simulink library "etherlab_lib_exp"  (Simulink 7.0)
undefined symbols (not defined in the file or in its folder): Address, catch_check
settings Model: Creator=rich  LastModifiedBy=ab  ExtModeAutoUpdateStatusClock=off

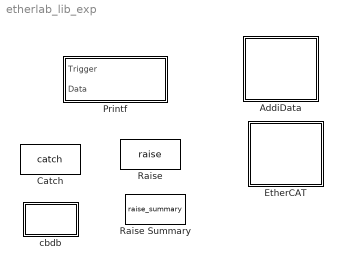
== system etherlab_lib_exp ==
  AddiData : Subsystem
  Catch : S-Function  InitFcn=catch_check(gcb,'CheckIds');  FunctionName=catch  Parameters=ErrId,dtype,Width,TSample  mask{ErrId=E10, dtype=boolean, TSample=0, Width=0, SrcPath=0, SrcCount=0}
      mask prompts: ErrId "Error Identifier"; dtype "Output Data Type Mode"; TSample "Sample Time (-1 inherited)"; SrcPath "Source Paths (Info only)"; SrcCount "Source Count"
      mask StyleString: edit,popup(double|single|int8|uint8|int16|uint16|int32|uint32|boolean|Inherit via back propagation),edit,edit,edit,edit
      mask CallbackString: catch_check(gcb,'CheckIds');|||||
      mask Display: fprintf('%s',ErrId);
  EtherCAT : Subsystem
  Printf : Subsystem  mask{format=0}
      mask prompts: format "Format String"
  Raise : S-Function  FunctionName=raise  Parameters=ErrId,ErrStr,TSample  mask{ErrId=E10, ErrStr=Voltage Too High, TSample=-1, DstPath=0, DstCount=0}
      mask prompts: ErrId "Error Identifier"; ErrStr "Error String"; TSample "Sample Time (-1 inherited)"; DstPath "Destination Paths"; DstCount "Destination Count"
      settings: CopyFcn=raise_check(gcb,'CheckCopy');
      mask CallbackString: raise_check(gcb,'CheckId');||||
      mask Display: fprintf('%s',ErrId);
  Raise Summary : S-Function  FunctionName=raise_summary  Parameters=ErrId,ErrStr,ErrSrc,DstPath  mask{ErrId=E1x, ErrStr=Voltage Too High, ErrSrc=E10, DstPath=0}
      mask prompts: ErrId "Error Identifier"; ErrStr "Error String"; ErrSrc "Error Sources"; DstPath "Destination Paths"
      settings: CopyFcn=raise_summary_check(gcb,'CheckCopy');
      mask Display: fprintf('%s\n%s',ErrId,ErrSrc);
  cbdb : Subsystem  LoadFcn=|  InitFcn=|  StartFcn=|  StopFcn=|  ClipboardFcn=|
      | if ~strcmp(gcs,'rtai_lib')
      | display('LoadFcn');       
      | end
      | if ~strcmp(gcs,'rtai_lib')
      | display('InitFcn');       
      | end
      | if ~strcmp(gcs,'rtai_lib')
      | display('StartFcn');      
      | end
      | if ~strcmp(gcs,'rtai_lib')
      | display('StopFcn');       
      | end
      | if ~strcmp(gcs,'rtai_lib')
      | display('ClipboardFcn');  
      | end
      settings: CopyFcn=|
      | if ~strcmp(gcs,'rtai_lib')
      | display('CopyFcn');
      | end
      settings: DeleteFcn=|
      | if ~strcmp(gcs,'rtai_lib')
      | display('DeleteFcn');
      | end
      settings: UndoDeleteFcn=|
      | if ~strcmp(gcs,'rtai_lib')
      | display('UndoDeleteFcn');
      | end
      settings: ModelCloseFcn=|
      | if ~strcmp(gcs,'rtai_lib')
      | display('ModelCloseFcn');
      | end
      settings: PreSaveFcn=|
      | if ~strcmp(gcs,'rtai_lib')
      | display('PreSaveFcn');
      | end
      settings: PostSaveFcn=|
      | if ~strcmp(gcs,'rtai_lib')
      | display('PostSaveFcn');
      | end
      settings: NameChangeFcn=|
      | if ~strcmp(gcs,'rtai_lib')
      | display('NameChangeFcn');
      | end
      settings: DestroyFcn=|
      | if ~strcmp(gcs,'rtai_lib')
      | display('DestroyFcn');
      | end
      settings: OpenFcn=|
      | if ~strcmp(gcs,'rtai_lib')
      | display('OpenFcn');
      | end
      settings: CloseFcn=|
      | if ~strcmp(gcs,'rtai_lib')
      | display('CloseFcn');
      | end
      settings: ParentCloseFcn=|
      | if ~strcmp(gcs,'rtai_lib')
      | display('ParentCloseFcn');
      | end
      settings: MoveFcn=|
      | if ~strcmp(gcs,'rtai_lib')
      | display('MoveFcn');
      | end
      mask Display: disp('Callback\nDebugger');

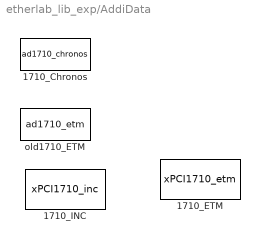
== system etherlab_lib_exp/AddiData ==
  1710_Chronos : S-Function  FunctionName=ad1710_chronos  Parameters=b_BoardHandle,b_ModuleNumber,b_ChronoMode,b_PCIInputClock,b_TimeUnit,ul_TimeOut,b_TimeoutUnit  mask{b_BoardHandle=0, b_ModuleNumber=0, b_ChronoMode=0, b_PCIInputClock=30MHz, b_TimeUnit=Microseconds, ul_TimeOut=0, b_TimeoutUnit=Micoseconds}
      mask prompts: b_BoardHandle "Board Handle"; b_ModuleNumber "Module Number"; b_ChronoMode "Chrono Mode"; b_PCIInputClock "PCI Input Clock"; b_TimeUnit "Time Unit"; ul_TimeOut "Timeout"; b_TimeoutUnit "Timeout Unit"
      mask StyleString: edit,popup(0|1|2|3),popup(0|1|2|3|4|5|6|7),popup(30MHz|33MHz|40MHz),popup(Nanoseconds|Microseconds|Milliseconds|Seconds|Minutes),edit,popup(Nanoseconds|Micoseconds|Milliseconds|Seconds|Minutes)
      mask Display:
      | fprintf('1710 Chrono\nB:%i M/d:%i',
      | b_BoardHandle,b_ModuleNumber);
  1710_ETM : S-Function  FunctionName=xPCI1710_etm  Parameters=device,module,clock_src,divisor,op_type,tsample  mask(Addi Data 1710 ETM){device=01:0A, module=0, clock_src=Internal 40MHz, divisor=1, op_type=double, scale=0, offset=0, tsample=0}
      mask prompts: device "PCI Device"; module "Module Number"; clock_src "Clock Source"; divisor "Clock Divisor"; op_type "Output Data Type"; scale "Output Full Scale"; offset "Output Offset"; tsample "Sampling Time (-1 inherited)"
      mask help: This block implements the Edge Triggered Timer Mode for the 1710 Addi Data timer card.
      mask init:
      | device = test_var(device);
      mask StyleString: edit,popup(0|1|2|3),popup(Internal 40MHz|PCI Bus 33/30Mhz),edit,popup(double|single|int8|uint8|int16|uint16|int32|uint32|boolean|Inherited via back propagation),edit,edit,edit
      mask Display:
      | fprintf('xPCI1710 ETM\nPCI: %s\nModule: %i',
      | device,module-1);
  1710_INC : S-Function  FunctionName=xPCI1710_inc  Parameters=device,module,mode,width,op_type,preset,tsample  mask(Addi Data 1710 INC){device=03:0E, module=0, mode=Quadruple, width=32-Bit, op_type=double, preset=off, tsample=0}
      mask prompts: device "PCI Device"; module "Module Number"; width "Counter Width"; op_type "Output Data Type"; preset "Preset Input"; tsample "Sampling Time (-1 inherited)"
      mask help: This block implements the Incremental Counter Mode for the 1710 Addi Data timer card.
      mask init:
      | device = test_var(device);
      mask StyleString: edit,popup(0|1|2|3),popup(Quadruple|Double|Simple|Direct),popup(32-Bit|16-Bit),popup(double|single|int8|uint8|int16|uint16|int32|uint32|boolean|Inherited via back propagation),checkbox,edit
      mask Display:
      | fprintf('xPCI1710 INC\nPCI: %s\nModule: %i',
      | device,module-1);
  old1710_ETM : S-Function  FunctionName=ad1710_etm  Parameters=b_BoardHandle,b_ModuleNumber,b_ClockSelection,b_TimingUnit,ul_Timing  mask(Addi Data 1710 ETM){b_BoardHandle=0, b_ModuleNumber=0, b_ClockSelection=PCI 30MHz, b_TimingUnit=Microseconds, ul_Timing=0}
      mask prompts: b_BoardHandle "Board Handle"; b_ModuleNumber "Module Number"; b_ClockSelection "Clock Selection"; b_TimingUnit "Timing Unit"; ul_Timing "Time Base"
      mask help:
      | This block implements the Edge Triggered Mode for the 1710 Addi Data timer card.
      |
      | Both counters are exported as a vector.
      mask StyleString: edit,popup(0|1|2|3),popup(PCI 30MHz|PCI 33MHz|Internal 40MHz),popup(Nanoseconds|Microseconds|Milliseconds),edit
      mask Display:
      | fprintf('1710 ETM\nB:%i M/d:%i',
      | b_BoardHandle,b_ModuleNumber);

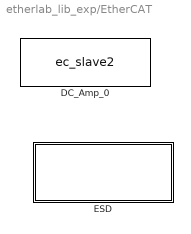
== system etherlab_lib_exp/EtherCAT ==
  DC_Amp_0 : S-Function  FunctionName=ec_slave2  Parameters=Address,config.SlaveConfig,config.SdoConfig,config.SoeConfig,config.IO,debug,tsample  mask(EL73x2){master=0, index=1, model=EL7332r00100000, dcmode=FreeRun/SM-Synchron, dccustom=[1 hex2dec('700') 0 0 0 0 0 0 0], max_current=[0 0], nom_current=[0 0], nom_volt=[0 0], resistance=[0 0], red_current_neg=[0 0], red_current_pos=[0 0], kp=[200 200], ki=[2 2], voltage_adjust_ch1=off, voltage_adjust_ch2=off, current_adjust_ch1=off, current_adjust_ch2=off, op_mode_ch1=Velocity direct, op_mode_ch2=Velocity direct, inv_dir_ch1=off, inv_dir_ch2=off, show_info_channels=off, datafield1_ch1=Coil Voltage, datafield2_ch1=Coil Current, datafield1_ch2=Coil Voltage, datafield2_ch2=Coil Current, show_digital_inputs=off, inv_input1_ch1=off, inv_input2_ch1=off, inv_input1_ch2=off, inv_input2_ch2=off, mode_input1_ch1=Normal Input, mode_input2_ch1=Normal Input, mode_input1_ch2=Normal Input, mode_input2_ch2=Normal Input, tsample=-1, debug=0, updatefcn=beckhoff_el73x2}
      mask prompts: index "Slave Index"; model "Device Model"; dcmode "DC Mode"; dccustom "DC Customized"; max_current "Max Motor Current in mA"; nom_current "Nominal Motor Currnet in mA"; nom_volt "Nominal Motor Voltage in mV"; resistance "Motor Resistance in 1/100 Ohm"; red_current_neg "Reduced Current (negative) in mA"; red_current_pos "Reduced Current (positive) in mA"; kp "Controller kp"; ki "Controller ki"; voltage_adjust_ch1 "Enable Voltage Adjustment Channel1"; voltage_adjust_ch2 "Enable Voltage Adjustment Channel2"; current_adjust_ch1 "Enable Current Adjustment Channel1"; current_adjust_ch2 "Enable Current Adjustment Channel2"; op_mode_ch1 "Operating Mode Channel1"; op_mode_ch2 "Operating Mode Channel2"; inv_dir_ch1 "Invert Motor direction Channel1"; inv_dir_ch2 "Invert Motor direction Channel2"; show_info_channels "Show Info Fields"; datafield1_ch1 "Info Field1 Channel 1"; datafield2_ch1 "Info Field2 Channel 2"; datafield1_ch2 "Info Field1 Channel 2"; datafield2_ch2 "Info Field2 Channel 2"; show_digital_inputs "Show Digital Inputs"; inv_input1_ch1 "Invert DI1 Channel1"; inv_input2_ch1 "Invert DI2 Channel1"; inv_input1_ch2 "Invert DI1 Channel2"; inv_input2_ch2 "Invert DI2 Channel2"; mode_input1_ch1 "Mode DI1 Channel1"; mode_input2_ch1 "Mode DI2 Channel1"; mode_input1_ch2 "Mode DI1 Channel2"; mode_input2_ch2 "Mode DI2 Channel2"; tsample "Sample Time (-1 for inherited)"
      mask help: Beckhoff 2 Channel DC Amplifier EL73x2
      mask init:
      | masterStr = '';
      | positionStr = '';
      | 
      | [Address masterStr positionStr] = getEtherCATAddress(gcb,master,index);
      | 
      | selection = beckhoff_el73x2('getmodel',model);
      | if isempty(selection)
      |     return;
      | end
      | 
      | func = selection{3};
      | 
      | device = beckhoff_el73x2('loaddescription',selection);
      | if isempty(device)
      |    return; 
      | end
      | 
      | 
      | %Prepare S-Funtion structure
      | 
      | config = beckhoff_el73x2('process',selection,device, ...
      |         max_current,nom_current,nom_volt,resistance, ...
      |         red_current_neg,red_current_pos, kp,ki,...
      |         voltage_adjust_ch1,current_adjust_ch1,...
      |         op_mode_ch1, inv_dir_ch1, ...
      |         datafield1_ch1,datafield2_ch1, ...
      |         inv_input1_ch1, inv_input2_ch1,...
      |         mode_input1_ch1, mode_input2_ch1,...
      |         voltage_adjust_ch2,current_adjust_ch2,...
      |         op_mode_ch2, inv_dir_ch2, ...
      |         datafield1_ch2,datafield2_ch2, ...
      |         inv_input1_ch2, inv_input2_ch2,...
      |         mode_input1_ch2, mode_input2_ch2,...
      |        show_digital_inputs, show_info_channels,...
      |        dcmode,dccustom ...
      |     );
      mask Help:
      | This block implements the EtherCAT 2 Channel DC Amplifier Terminal EL73x2.
      | <p/>
      | The block input and output depends generally on the configured functionality. Please read the Terminal documentation.
      | <p/>
      | The following Terminals are supported:
      | <center>
      | <table width="80%">
      | <tr><td>EL7332</td><td></td></tr>
      | </table>
      | </center>
      | <p/>
      | 
      | 
      | 
      | <h4>Inputs:</h4>
      | Every Block Input is a 2-element Vector ([Channel1 Channel2])
      | <p>
      | Following Inputs exists:
      | <ul>
      | <li> Enable</li>
      | <li> Reset</li>
      | <li> Reduce Torque</li>
      | <li> Setpoint Current</li>
      | <ul/>
      | <h4>Outputs:</h4>
      | Every Block Output is a 2-element Vector ([Channel1 Channel2])
      | <p>
      | Following Outputs exists:
      | <ul>
      | <li> Ready to Enable </li>
      | <li> Ready </li>
      | <li> Warning</li>
      | <li> Error</li>
      | <li> Digital Input 1 (optional)</li>
      | <li> Digital Input 2 (optional)</li>
      | <li> Info Channel 1 (optional)</li>
      | <li> Info Channel 2 (optional)</li>
      | </ul>
      | Choose and set the following options:
      | <h4>Master:</h4>
      | Set the EtherCAT Master of this terminal.
      | 
      | <h4>Slave Index:</h4>
      | Set the EtherCAT slave index. Following address formats are allowed:
      | <ol>
      | <li> Absolute addressing: a scalar number <<b><tt>n</tt></b>> representing the (zero based) absolute position in the bus.
      | <li> SSId addressing: the Secondary Slave (or 'Alias') Addressing has the form <<b><tt>[alias position]</tt></b>> where <b><tt>alias</tt></b> is the Secondary Slave Id of the EtherCAT slave and <b><tt>position</tt></b> is the offset after the slave with the given <b><tt>alias</tt></b>. The SSId has to be preprogrammed into the slave with other service tools (see 'ethercat alias --help').
      | </ol>
      | 
      | <h4>Device Model:</h4>
      | Choose the device at the Indexed position of the master.
      | 
      | <h4>DC Mode:</h4>
      | Choose the DC Mode for the module.
      | 
      | <h4>DC Customer:</h4>
      | Do customized DC Settings in a vector
      | <<b><tt>[Index AssignActivate cycletimesync0 factor0 cycletimeshift0 input0 cycletimesync1 factor1 cylcetimeshift1]</tt></b>>
      | 
      | <ul>
      | <li><<b><tt>Index:</tt></b>> preload index from XML desctiption, to get the oversampling configuration from an existing DC-mode.
      | <li><<b><tt>AssignActivate:</tt></b>> Value for DC-mode setting
      | <li><<b><tt>cycletimesync0:</tt></b>> CycletimeSync0 Value
      | <li><<b><tt>factor0:</tt></b>> 1 or 0. If factor0 equals one the cycletimesync0 value is internally set to the process cycletime.
      | <li><<b><tt>cycletimeshift0:</tt></b>> Cycletimeshift0 Value
      | <li><<b><tt>input0:</tt></b>> 1 or 0. If inpot0 equals one the Slave is synced on the input event
      | <li><<b><tt>cycletimesync1:</tt></b>> CycletimeSync1 Value
      | <li><<b><tt>factor1:</tt></b>> 1 or 0. If factor1 equals one the cycletimesync1 value is internally set to the process cycletime.
      | <li><<b><tt>cylcetimeshift1:</tt></b>> Cycletimeshift1 Value
      | </ul>
      | 
      | <h4>Max Motor Current in mA:</h4>
      | Maximal Motor Current in mA. Value has to be a 2 element vector: [0 0] ([Channel1 Channe2])
      | 
      | <h4>Nominal Motor Current in mA:</h4>
      | Nominal Motor Current in mA. Value has to be a 2 element vector: [0 0] ([Channel1 Channe2])
      | 
      | <h4>Nominal Motor Voltage in mV:</h4>
      | Nominal Motor Voltage in mV. Value has to be a 2 element vector: [0 0] ([Channel1 Channe2])
      | 
      | <h4>Motor Resistance in 1/100 Ohm:</h4>
      | Motor Resistance in 1/100 Ohm. Value has to be a 2 element vector: [0 0] ([Channel1 Channe2])
      | 
      | <h4>Reduced Current (negative) in mA:</h4>
      | Reduced Current Value in negative Direction. Value has to be a 2 element vector: [0 0] ([Channel1 Channe2])
      | 
      | <h4>Reduced Current (positive) in mA:</h4>
      | Reduced Current Value in positive Direction. Value has to be a 2 element vector: [0 0] ([Channel1 Channe2])
      | 
      | <h4>Controller kp:</h4>
      | Motor Controller Setting for kp. Value has to be a 2 element vector: [0 0] ([Channel1 Channe2])
      | 
      | <h4>Controller ki:</h4>
      | Motor Controller Setting for ki. Value has to be a 2 element vector: [0 0] ([Channel1 Channe2])
      | 
      | <h4>Enable Voltage Adjustment Channel[1,2]:</h4>
      | Activates Voltage swing compensation for Channel [1,2].
      | 
      | <h4>Enable Current Adjustment Channel[1,2]:</h4>
      | Activates RxI compensation for Channel [1,2].
      | 
      | <h4>Operating Mode Channel[1,2]:</h4>
      | Select Operating Mode for Channel [1,2]. Actually only Velocity direct is implemeneted.
      | 
      | <h4>Invert Motor direction Channel[1,2]:</h4>
      | Invert Rotyting direction for Channel [1,2].
      | 
      | <h4>Show Info Fields:</h4>
      | Enable or Disable the Output of the configurable PDO Outputs.
      | 
      | <h4>Info Field[X=1,2] Channel[Y=1,2]</h4>
      | Configure the output info fields. 2 Info outputs per channel exists.
      | Actually only the selection of State, Current and Voltage are supported.
      | 
      | <h4>Show Digital Inputs:</h4>
      | Enable or Disable the Output of the digital inputs.
      | 
      | <h4>Invert DI[X=1,2] Channel[Y=1,2]</h4>
      | Invert the digital input. 2  digital inputs per channel exists.
      | 
      | <h4>Mode DI[X=1,2] Channel[Y=1,2]</h4>
      | Working mode of the digital input. 2  digital inputs per channel exists.
      | Normal input or Hardware enable are available.
      | 
      | <p>
      | To get further information for parameter configuration, please read the terminal documentation.
      | <p>
      | Set the <b>Sample Time</b> for the block. <tt>0</tt> is continuous sample time (runs at the model's base rate). Setting <tt>-1</tt> will try to set the time using back propagation.
      mask StyleString: edit,edit,popup(EL7332r00100000|EL7332r00110000),popup(FreeRun/SM-Synchron|DC-Synchron|DC-Customized),edit,edit,edit,edit,edit,edit,edit,edit,edit,checkbox,checkbox,checkbox,checkbox,popup(Automatic|Velocity direct|Velocity controller|Position controller),popup(Automatic|Velocity direct|Velocity controller|Position controller),checkbox,checkbox,checkbox,popup(Status word|Coil Voltage|Coil Current),popup(Status word|Coil Voltage|Coil Current),popup(Status word|Coil Voltage|Coil Current),popup(Status word|Coil Voltage|Coil Current),checkbox,checkbox,checkbox,checkbox,checkbox,popup(Normal Input|Hardware Enable),popup(Normal Input|Hardware Enable),popup(Normal Input|Hardware Enable),popup(Normal Input|Hardware Enable),edit,edit,edit
      mask CallbackString: ||beckhoff_el73x2('model');|beckhoff_el73x2('dc');||||||||||||||||||||||||||||||||||
      mask Display:
      | fprintf('%s\n%s \nM:%s Idx:%s',...
      |     model,func,masterStr,positionStr)
  ESD : Subsystem
      mask Display: image(imread('ESD.png'))

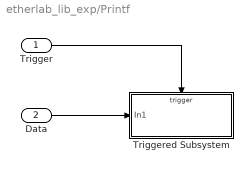
== system etherlab_lib_exp/Printf ==
  Trigger : Inport  OutDataType=sfix(16)  OutScaling=2^0
  Data : Inport  Port=2  OutDataType=sfix(16)  OutScaling=2^0
  Triggered Subsystem : Subsystem  TreatAsAtomicUnit=on
  wires:
  Trigger/1 -> Triggered Subsystem/Trigger
  Data/1 -> Triggered Subsystem/1(In1)

== system etherlab_lib_exp/cbdb ==

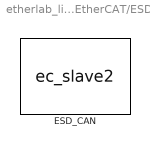
== system etherlab_lib_exp/EtherCAT/ESD ==
  ESD_CAN : S-Function  FunctionName=ec_slave2  Parameters=Address,conf.SlaveConfig,conf.SdoConfig,conf.SoeConfig,conf.IO,debug,tsample  mask(ESD EtherCAT CAN Gateway){master=0, index=1, model=CANr00000000, numberrx=1, numbertx=1, isext=off, baudrate=500, rxfilter=[], nodeadr=1, tsample=-1, debug=0, updatefcn=esd_cangateway}
      mask prompts: index "Slave Index"; model "Device Model"; numberrx "MailboxSize RX"; numbertx "MailboxSize TX"; isext "Extended ID"; baudrate "Baudrate in kBit/s"; rxfilter "RX Filter IDs"; nodeadr "Node ID"; tsample "Sample Time (-1 for inherited)"
      mask help:
      | ESD EtherCAT
      | CAN Gateway
      mask init:
      | masterStr = '';
      | positionStr = '';
      | [Address masterStr positionStr] = getEtherCATAddress(gcb,master,index);
      | 
      | selection = esd_cangateway('getmodel',model);
      | if isempty(selection)
      |     return;
      | end
      | 
      | func = selection{3};
      | 
      | device = esd_cangateway('loaddescription',selection);
      | if isempty(device)
      |    return; 
      | end
      | 
      | 
      | %Prepare S-Funtion structure
      | 
      | conf = esd_cangateway('process',selection,device,numberrx,numbertx,isext,baudrate,rxfilter,nodeadr);
      mask Help:
      | This block generically implements the ESD EtherCAT CAN Gateway.
      | 
      | <p/>
      | The following Terminals are supported:
      | <center>
      | <table width="80%">
      | <tr><td>CAN</td><td> EtherCAT CAN Gateway</td></tr>
      | </table>
      | </center>
      | <h3> Inputs / Outputs</h3>
      | <h4>Inputs</h4>
      | There are two block inputs.
      | <p>
      | First port the static informations (Vector of 3x UINT16)
      | <ul>
      | <li> TX-Counter: Control send counter </li>
      | <li> RX-Counter: Control recieve counter </li>
      | <li> No Messages: Number of messages to send</li>
      | </ul>
      | <p>
      | Second port the message vector (Vector XxUINT8)
      | The size of the vector depends on
      | <ul>
      | <li> Size of the configured TX-Message Queque
      | <li> Messages are extended (31 Bit ID) or normal (11 Bit ID)
      | </ul>
      | <p>
      | The vector size is calculated to
      | <ul>
      | <li>(11Bit ID) No Messages x 12 Byte
      | <li>(31 Bit ID) No Messages x 16 Byte
      | </ul>
      | 
      | 
      | <h3> Inputs / Outputs</h3>
      | <h4>Outputs</h4>
      | There are two block outputs.
      | <p>
      | First port the static informations (Vector of 4x UINT16)
      | <ul>
      | <li> TX-Counter: Control send counter </li>
      | <li> RX-Counter: Control recieve counter </li>
      | <li> No Messages: Number of messages to send</li>
      | <li> Transaction No: last accessed transaction No
      | </ul>
      | <p>
      | Second port the message vector (Vector XxUINT8)
      | The size of the vector depends on
      | <ul>
      | <li> Size of the configured RX-Message Queque
      | <li> Messages are extended (31 Bit ID) or normal (11 Bit ID)
      | </ul>
      | <p>
      | The vector size is calculated to
      | <ul>
      | <li>(11Bit ID) No Messages x 10 Byte
      | <li>(31 Bit ID) No Messages x 14 Byte
      | </ul>
      | 
      | <p/>
      | Choose and set the following options:
      | <h4>Master:</h4>
      | Set the EtherCAT Master of this terminal.
      | 
      | <h4>Slave Index:</h4>
      | Set the EtherCAT slave index. Following address formats are allowed:
      | <ol>
      | <li> Absolute addressing: a scalar number <<b><tt>n</tt></b>> representing the (zero based) absolute position in the bus.
      | <li> SSId addressing: the Secondary Slave (or 'Alias') Addressing has the form <<b><tt>[alias position]</tt></b>> where <b><tt>alias</tt></b> is the Secondary Slave Id of the EtherCAT slave and <b><tt>position</tt></b> is the offset after the slave with the given <b><tt>alias</tt></b>. The SSId has to be preprogrammed into the slave with other service tools (see 'ethercat alias --help').
      | </ol>
      | 
      | 
      | 
      | <h4>Device Model:</h4>
      | Choose the device at the Indexed position of the master.
      | 
      | <h4>MailboxSize RX / TX</h4>
      | Configure the RX/TX Queque size of the Slave.
      | 
      | 
      | <h4>Extended ID</h4>
      | Enables Extended (31 Bit) CAN ID handling.
      | 
      | 
      | <h4>Baudrate</h4>
      | Configure the CAN Baudrate.
      | 
      | 
      | <h4>RX Filter IDs</h4>
      | Configure the RX Filter ID. Only the selected IDs will be accessed on the CAN Bus. If the vector is empty, all messages are prceded.
      | The vector has to be [1 2 3 4 5].
      | 
      | <h4>Node ID</h4>
      | Configure the CAN node id.
      | 
      | <p>
      | Set the <b>Sample Time</b> for the block. <tt>0</tt> is continuous sample time (runs at the model's base rate). Setting <tt>-1</tt> will try to set the time using back propagation.
      mask StyleString: edit,edit,popup(CANr00000000),edit,edit,checkbox,popup(1000|800|500|250|125|100|50),edit,edit,edit,edit,edit
      mask Display:
      | fprintf('ESD EtherCAT\n%s\n%s\nM:%s Idx:%s',...
      |     model,func,masterStr,positionStr)

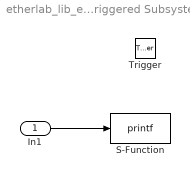
== system etherlab_lib_exp/Printf/Triggered Subsystem ==
  In1 : Inport  OutDataType=sfix(16)  OutScaling=2^0
  Trigger : TriggerPort
  S-Function : S-Function  FunctionName=printf  Parameters=format
  wires:
  In1/1 -> S-Function/1
